simulink model "FINALMAGLEV"  (R2023b)
settings: Solver=VariableStepAuto  StartTime=0.0  StopTime=5  RelTol=1e-3
values from neighbouring files (symbols this model uses):
  A = [0 1 0 ... (first row only)    [magneticlevitation.m]
  B = [0; 0; 100]    [magneticlevitation.m]
  C = [1 0 0]    [magneticlevitation.m]
  K = acker(A_bar, B_bar, cl_poles)    [magneticlevitation.m]
settings Model: LastModifiedBy=91798

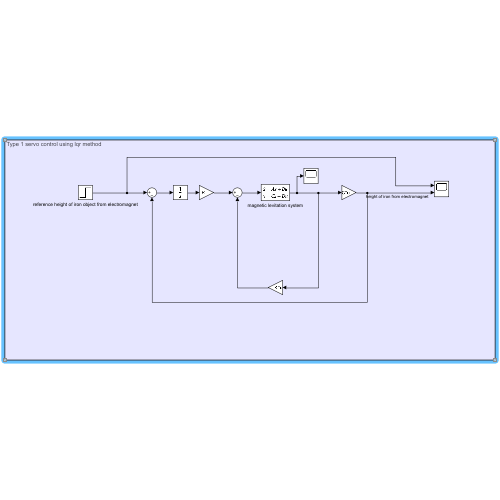
[thumbnail: Simulink's stored preview of the top-level diagram]
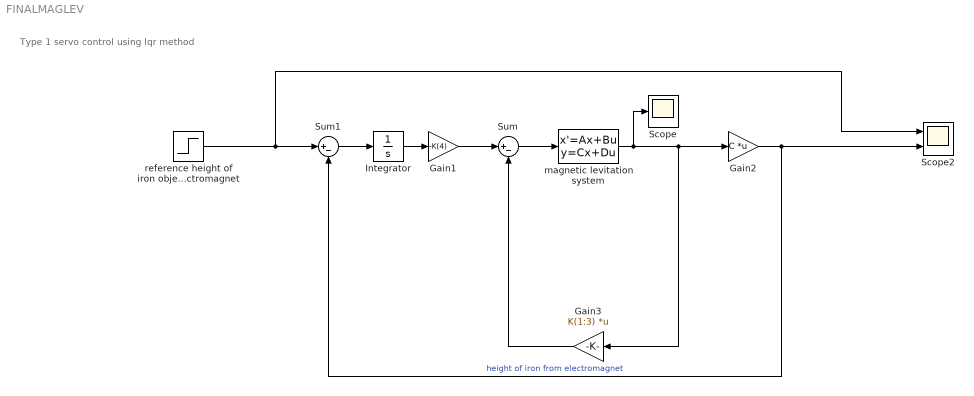
== system FINALMAGLEV ==
  note: Type 1 servo control using lqr method
  Gain1 : Gain  Gain=-K(4)
  Gain2 : Gain  Gain=C  Multiplication=Matrix(K*u)
  Gain3 : Gain  Gain=K(1:3)  Multiplication=Matrix(K*u)
  Integrator : Integrator
  Scope : Scope
  Scope2 : Scope  NumInputPorts=2
  Sum : Sum  Inputs=|+-
  Sum1 : Sum  Inputs=|+-
  magnetic levitation system : StateSpace  A=A  B=B  C=eye(3)  D=zeros(3,1)  InitialCondition=0
  reference height of iron object from electromagnet : Step  Time=2.5  SampleTime=0
  wires:
  Sum/1 -> magnetic levitation system/1
  Gain1/1 -> Sum/1
  magnetic levitation system/1 -> Scope/1, Gain3/1, Gain2/1
  Integrator/1 -> Gain1/1
  Sum1/1 -> Integrator/1
  Gain2/1 -> Scope2/2, Sum1/2  "height of iron from electromagnet"
  reference height of iron object from electromagnet/1 -> Scope2/1, Sum1/1
  Gain3/1 -> Sum/2
